simulink model "RefModel_compass_out2"  (R2019b)
settings: Solver=FixedStepDiscrete  StartTime=0.0  StopTime=35  FixedStep=0.1  RelTol=1e-3
values from neighbouring files (symbols this model uses):
  ax = double(typecast(uint8(temp),'single')')/1*1.0000000000    [V1000_decode_auto.m]
  ay = double(typecast(uint8(temp),'single')')/1*1.0000000000    [V1000_decode_auto.m]
  az = double(typecast(uint8(temp),'single')')/1*1.0000000000    [V1000_decode_auto.m]
  gx = double(typecast(uint8(temp),'single')')/1*1.0000000000    [V1000_decode_auto.m]
  gy = double(typecast(uint8(temp),'single')')/1*1.0000000000    [V1000_decode_auto.m]
  gz = double(typecast(uint8(temp),'single')')/1*1.0000000000    [V1000_decode_auto.m]
undefined symbols (not defined in the file or in its folder): ax_f, ay_f, az_f, gx_f, gy_f, gz_f, HD, mag2_xx, mag2_yx, mag2_zx, time_algo, time_imu, time_mag
libraries: simulink x1, aerolibgravity2 x1
settings Model: Creator=sl  LastModifiedBy=a4327
settings OptimizationCC: DefaultParameterBehavior=Inlined  UseDivisionForNetSlopeComputation=on  GainParamInheritBuiltInType=on  UseFloatMulNetSlope=on  InlineInvariantSignals=on  PassReuseOutputArgsAs=Individual arguments  ZeroExternalMemoryAtStartup=off  ZeroInternalMemoryAtStartup=off  NoFixptDivByZeroProtection=on  EfficientFloat2IntCast=on  LifeSpan=1  OptimizeBlockOrder=speed  DifferentSizesBufferReuse=on  EfficientTunableParamExpr=on
settings DebuggingCC: ParameterTunabilityLossMsg=error  ArithmeticOperatorsInVariantConditions=warning
settings HardwareCC: ProdBitPerPointer=32  ProdBitPerSizeT=32  ProdBitPerPtrDiffT=32  ProdLargestAtomicFloat=None  ProdWordSize=32  ProdLongLongMode=on  ProdHWDeviceType=Custom Processor->Custom Processor
settings SFSimCC: MATLABDynamicMemAlloc=off  CustomCodeUndefinedFunction=UseInterfaceOnly
settings RTWCC: SystemTargetFile=ert.tlc  TemplateMakefile=ert_default_tmf  GenerateReport=on  IncludeHyperlinkInReport=on  LaunchReport=on  GenerateTraceInfo=on  GenerateTraceReport=on  GenerateTraceReportSl=on  GenerateTraceReportSf=on  GenerateTraceReportEml=on  GenerateCodeMetricsReport=on
settings CodeAppCC: ForceParamTrailComments=on  IgnoreCustomStorageClasses=off  OperatorAnnotations=on  SimulinkDataObjDesc=on  SFDataObjDesc=on  CustomSymbolStrGlobalVar=rt$N$M  CustomSymbolStrType=$N$M  CustomSymbolStrFcn=$N$M$F  CustomSymbolStrMacro=$N$M  InsertBlockDesc=on
settings ERTTargetCC: TargetLangStandard=C99 (ISO)  GenerateSampleERTMain=on  IncludeMdlTerminateFcn=off  CombineSignalStateStructs=on  SupportAbsoluteTime=off  SupportComplex=off  SupportNonInlinedSFcns=on  InlinedParameterPlacement=NonHierarchical  ERTCustomFileTemplate=example_file_process.tlc  ERTFilePackagingFormat=CompactWithDataFile

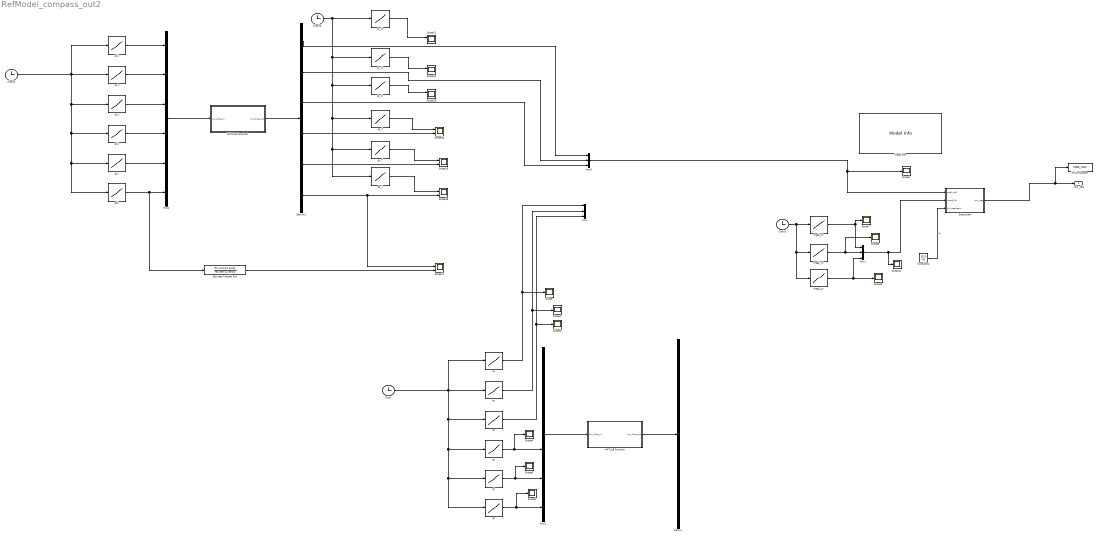
== system RefModel_compass_out2 ==
  Clock{,1..3} (4 alike) : Clock
  Constant2 : Constant  Value=[0 0 0]
  Demux : Demux  Outputs=6
  Demux1 : Demux  Outputs=6
  Discrete Transfer Fcn : DiscreteTransferFcn  Numerator=ftz.num{1:end}  Denominator=ftz.den{1:end}
  MATLAB Function : MATLAB Function  TreatAsAtomicUnit=on
  MATLAB Function1 : MATLAB Function  TreatAsAtomicUnit=on
  Model Info : simulink/Model-Wide Utilities/Model Info  Frame=on  DisplayStringWithTags=|  HorizontalTextAlignment=Left  LeftAlignmentValue=0.02
      | %<ModelVersion>
      | %<LastModificationDate>
      | 
      | Body Coordinate: forward - right - down
      | Navigation Coordinate: NED
      | 
      | input:
      | 	accB_ms2:  1x3  m/s^2
      | 	magB_Gs:   1x3  Gs
      | 	LLA_degdegm(lat,lon,height): 1x3 deg,deg,m  
      | output:
      | 	yaw_deg: 1x1 deg
  Mux : Mux  Inputs=3
  Mux1 : Mux  Inputs=3
  Mux2 : Mux  Inputs=6
  Mux3 : Mux  Inputs=3
  Mux4 : Mux  Inputs=6
  Scope{,1..10} (11 alike) : Scope
  Scope{11..17} (7 alike) : Scope  NumInputPorts=2
  Subsystem : Subsystem
  To Workspace : ToWorkspace  VariableName=MAG_YAW  SampleTime=-1
  ax : Lookup_n-D  NumberOfTableDimensions=1  BreakpointsForDimension1=time_imu  Table=ax  InternalRulePriority=Speed  RndMeth=Simplest  InputSameDT=on
  ax1 : Lookup_n-D  NumberOfTableDimensions=1  BreakpointsForDimension1=time_imu  Table=ax  InternalRulePriority=Speed  RndMeth=Simplest  InputSameDT=on
  ax_f1 : Lookup_n-D  NumberOfTableDimensions=1  BreakpointsForDimension1=time_algo  Table=ax_f  InternalRulePriority=Speed  RndMeth=Simplest  InputSameDT=on
  ay : Lookup_n-D  NumberOfTableDimensions=1  BreakpointsForDimension1=time_imu  Table=ay  InternalRulePriority=Speed  RndMeth=Simplest  InputSameDT=on
  ay1 : Lookup_n-D  NumberOfTableDimensions=1  BreakpointsForDimension1=time_imu  Table=ay  InternalRulePriority=Speed  RndMeth=Simplest  InputSameDT=on
  ay_f1 : Lookup_n-D  NumberOfTableDimensions=1  BreakpointsForDimension1=time_algo  Table=ay_f  InternalRulePriority=Speed  RndMeth=Simplest  InputSameDT=on
  az : Lookup_n-D  NumberOfTableDimensions=1  BreakpointsForDimension1=time_imu  Table=az  InternalRulePriority=Speed  RndMeth=Simplest  InputSameDT=on
  az1 : Lookup_n-D  NumberOfTableDimensions=1  BreakpointsForDimension1=time_imu  Table=az  InternalRulePriority=Speed  RndMeth=Simplest  InputSameDT=on
  az_f1 : Lookup_n-D  NumberOfTableDimensions=1  BreakpointsForDimension1=time_algo  Table=az_f  InternalRulePriority=Speed  RndMeth=Simplest  InputSameDT=on
  gx : Lookup_n-D  NumberOfTableDimensions=1  BreakpointsForDimension1=time_imu  Table=gx  InternalRulePriority=Speed  RndMeth=Simplest  InputSameDT=on
  gx1 : Lookup_n-D  NumberOfTableDimensions=1  BreakpointsForDimension1=time_imu  Table=gx  InternalRulePriority=Speed  RndMeth=Simplest  InputSameDT=on
  gx_f : Lookup_n-D  NumberOfTableDimensions=1  BreakpointsForDimension1=time_algo  Table=gx_f  InternalRulePriority=Speed  RndMeth=Simplest  InputSameDT=on
  gy : Lookup_n-D  NumberOfTableDimensions=1  BreakpointsForDimension1=time_imu  Table=gy  InternalRulePriority=Speed  RndMeth=Simplest  InputSameDT=on
  gy1 : Lookup_n-D  NumberOfTableDimensions=1  BreakpointsForDimension1=time_imu  Table=gy  InternalRulePriority=Speed  RndMeth=Simplest  InputSameDT=on
  gy_f : Lookup_n-D  NumberOfTableDimensions=1  BreakpointsForDimension1=time_algo  Table=gy_f  InternalRulePriority=Speed  RndMeth=Simplest  InputSameDT=on
  gz : Lookup_n-D  NumberOfTableDimensions=1  BreakpointsForDimension1=time_imu  Table=gz  InternalRulePriority=Speed  RndMeth=Simplest  InputSameDT=on
  gz1 : Lookup_n-D  NumberOfTableDimensions=1  BreakpointsForDimension1=time_imu  Table=gz  InternalRulePriority=Speed  RndMeth=Simplest  InputSameDT=on
  gz_f : Lookup_n-D  NumberOfTableDimensions=1  BreakpointsForDimension1=time_algo  Table=gz_f  InternalRulePriority=Speed  RndMeth=Simplest  InputSameDT=on
  mag2_xx : Lookup_n-D  NumberOfTableDimensions=1  BreakpointsForDimension1=time_mag  Table=mag2_xx  InternalRulePriority=Speed  RndMeth=Simplest  InputSameDT=on
  mag2_yx : Lookup_n-D  NumberOfTableDimensions=1  BreakpointsForDimension1=time_mag  Table=mag2_yx  InternalRulePriority=Speed  RndMeth=Simplest  InputSameDT=on
  mag2_zx : Lookup_n-D  NumberOfTableDimensions=1  BreakpointsForDimension1=time_mag  Table=mag2_zx  InternalRulePriority=Speed  RndMeth=Simplest  InputSameDT=on
  yaw_deg : Outport
  wires:
  Mux3/1 -> Scope1/1, Subsystem/1(accB_ms2)
  Constant2/1 -> Subsystem/3(LLA_degdegm)  "lla"
  Subsystem/1(yaw_deg) -> To Workspace/1, yaw_deg/1
  Clock1/1 -> mag2_zx/1, mag2_yx/1, mag2_xx/1
  gy/1 -> Scope5/1, Mux2/5
  gz/1 -> Scope6/1, Mux2/6
  Mux2/1 -> MATLAB Function/1(imu_filter_in)
  Clock/1 -> gz/1, gy/1, gx/1, az/1, ax/1, ay/1
  gx/1 -> Scope4/1, Mux2/4
  MATLAB Function/1(imu_filter_out) -> Demux/1
  mag2_yx/1 -> Scope8/1, Mux1/2
  mag2_xx/1 -> Scope7/1, Mux1/1
  mag2_zx/1 -> Scope9/1, Mux1/3
  Mux1/1 -> Scope10/1, Subsystem/2(magB_Gs)
  ax/1 -> Mux/1, Scope/1
  ay/1 -> Mux/2, Scope2/1
  az/1 -> Mux/3, Scope3/1
  gz_f/1 -> Scope16/1
  ay1/1 -> Mux4/2
  gx_f/1 -> Scope14/1
  ax1/1 -> Mux4/1
  Demux1/2 -> Mux3/2
  Clock3/1 -> gz_f/1, gy_f/1, gx_f/1, az_f1/1, ay_f1/1, ax_f1/1
  Demux1/6 -> Scope17/1, Scope16/2
  Demux1/5 -> Scope15/2
  Demux1/3 -> Mux3/3
  gy_f/1 -> Scope15/1
  Mux4/1 -> MATLAB Function1/1(imu_filter_in)
  ay_f1/1 -> Scope12/1
  gx1/1 -> Mux4/4
  Clock2/1 -> gz1/1, gy1/1, gx1/1, az1/1, ax1/1, ay1/1
  ax_f1/1 -> Scope11/1
  gz1/1 -> Discrete Transfer Fcn/1, Mux4/6
  Demux1/4 -> Scope14/2
  Demux1/1 -> Mux3/1
  az1/1 -> Mux4/3
  gy1/1 -> Mux4/5
  MATLAB Function1/1(imu_filter_out) -> Demux1/1
  az_f1/1 -> Scope13/1
  Discrete Transfer Fcn/1 -> Scope17/2

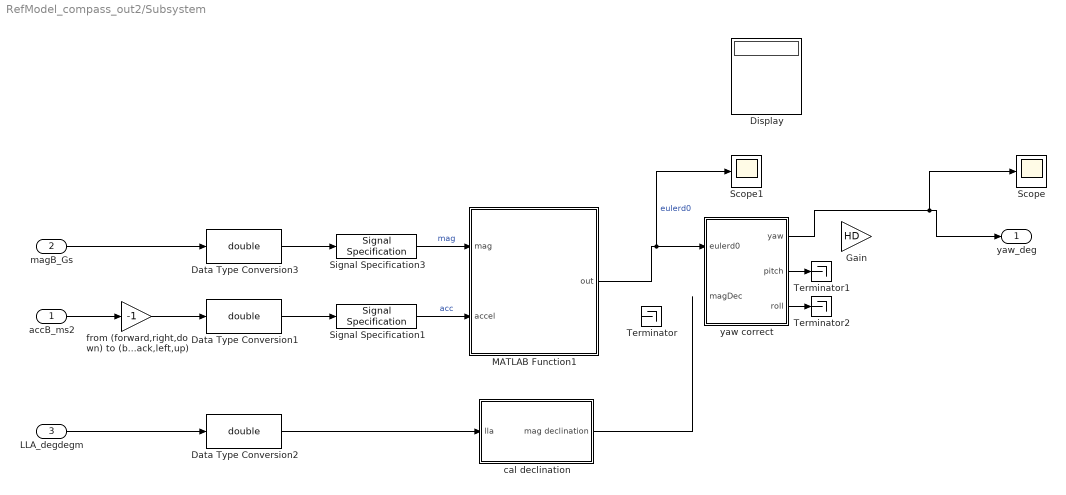
== system RefModel_compass_out2/Subsystem ==
  accB_ms2 : Inport  PortDimensions=[1,3]
  magB_Gs : Inport  Port=2  PortDimensions=[1,3]
  LLA_degdegm : Inport  Port=3  PortDimensions=[1,3]
  Data Type Conversion1 : DataTypeConversion  OutDataTypeStr=double
  Data Type Conversion2 : DataTypeConversion  OutDataTypeStr=double
  Data Type Conversion3 : DataTypeConversion  OutDataTypeStr=double
  Display : Display
  Gain : Gain  Gain=HD
  MATLAB Function1 : MATLAB Function  TreatAsAtomicUnit=on
  Scope : Scope
  Scope1 : Scope
  Signal Specification1 : SignalSpecification  Dimensions=[1,3]
  Signal Specification3 : SignalSpecification  Dimensions=[1,3]
  Terminator : Terminator
  Terminator1 : Terminator
  Terminator2 : Terminator
  cal declination : Subsystem
  from (forward,right,down) to (back,left,up) : Gain  Gain=-1
  yaw correct : Subsystem
  yaw_deg : Outport
  wires:
  from (forward,right,down) to (back,left,up)/1 -> Data Type Conversion1/1
  Signal Specification3/1 -> MATLAB Function1/1(mag)  "mag"
  yaw correct/2(pitch) -> Terminator1/1
  Data Type Conversion1/1 -> Signal Specification1/1
  Data Type Conversion3/1 -> Signal Specification3/1
  magB_Gs/1 -> Data Type Conversion3/1
  accB_ms2/1 -> from (forward,right,down) to (back,left,up)/1
  yaw correct/3(roll) -> Terminator2/1
  Signal Specification1/1 -> MATLAB Function1/2(accel)  "acc"
  cal declination/1(mag declination) -> ?
  Data Type Conversion2/1 -> cal declination/1(lla)
  LLA_degdegm/1 -> Data Type Conversion2/1
  MATLAB Function1/1(out) -> Scope1/1, yaw correct/1(eulerd0)  "eulerd0"
  yaw correct/1(yaw) -> Scope/1, yaw_deg/1

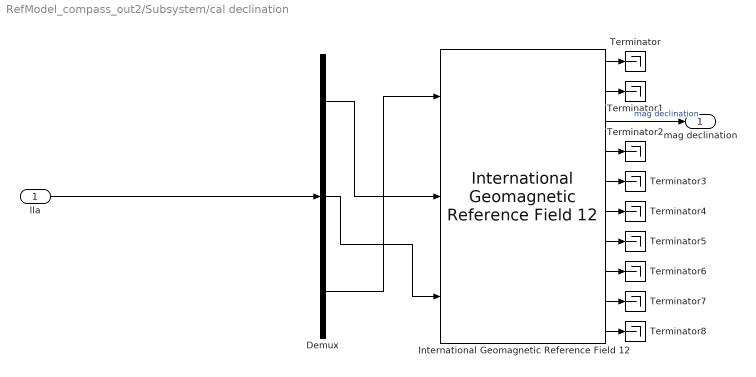
== system RefModel_compass_out2/Subsystem/cal declination ==
  lla : Inport
  Demux : Demux  Outputs=3
  International Geomagnetic Reference Field 12 : aerolibgravity2/International Geomagnetic Reference Field 12  units=Metric (MKS)  time_in=off  month=December  day=20  year=2019  action=None  sv_out=on
      settings: SourceProductName=Aerospace Blockset  SourceProductBaseCode=AE
  Terminator{,1..8} (9 alike) : Terminator
  mag declination : Outport
  wires:
  Demux/3 -> International Geomagnetic Reference Field 12/1
  Demux/1 -> International Geomagnetic Reference Field 12/2
  International Geomagnetic Reference Field 12/9 -> Terminator7/1
  International Geomagnetic Reference Field 12/10 -> Terminator8/1
  International Geomagnetic Reference Field 12/4 -> Terminator2/1
  International Geomagnetic Reference Field 12/1 -> Terminator/1
  Demux/2 -> International Geomagnetic Reference Field 12/3
  International Geomagnetic Reference Field 12/2 -> Terminator1/1
  International Geomagnetic Reference Field 12/3 -> mag declination/1  "mag declination"
  International Geomagnetic Reference Field 12/5 -> Terminator3/1
  International Geomagnetic Reference Field 12/6 -> Terminator4/1
  International Geomagnetic Reference Field 12/8 -> Terminator6/1
  International Geomagnetic Reference Field 12/7 -> Terminator5/1
  lla/1 -> Demux/1

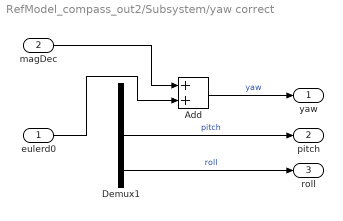
== system RefModel_compass_out2/Subsystem/yaw correct ==
  eulerd0 : Inport
  magDec : Inport  Port=2
  Add : Sum
  Demux1 : Demux  Outputs=3
  yaw : Outport
  pitch : Outport  Port=2
  roll : Outport  Port=3
  wires:
  magDec/1 -> Add/1
  Demux1/2 -> pitch/1  "pitch"
  Demux1/3 -> roll/1  "roll"
  eulerd0/1 -> Add/2
  Add/1 -> yaw/1  "yaw"

== matlab function RefModel_compass_out2/MATLAB Function1 ==
  data: imu_filter_in input; imu_filter_out output
function imu_filter_out = imu_filter(imu_filter_in)
% ftz.num{1:end}
% ftz.den{1:end}
% persistent
persistent imu_filter_in_buff
persistent imu_filter_out_buff
    if isempty(imu_filter_in_buff)
        imu_filter_in_buff = zeros(3,6);
    end
    if isempty(imu_filter_out_buff)
        imu_filter_out_buff = zeros(3,6);
    end 
    
    

imu_filter_in_buff(1,:)=imu_filter_in_buff(2,:);
imu_filter_in_buff(2,:)=imu_filter_in_buff(3,:);
imu_filter_in_buff(3,:)=imu_filter_in;
imu_filter_out_buff(1,:)=imu_filter_out_buff(2,:);
imu_filter_out_buff(2,:)=imu_filter_out_buff(3,:);
% imu_filter_out=imu_filter_in_buff(3,:)*0.1287+imu_filter_in_buff(2,:)*0.2574+imu_filter_in_buff(1,:)*0.1287-imu_filter_out_buff(2,:)*- 0.7613-imu_filter_out_buff(1,:)*0.276;
imu_filter_out=imu_filter_in_buff(3,:)*0.008771+imu_filter_in_buff(2,:)*0.01754+imu_filter_in_buff(1,:)*0.008771-imu_filter_out_buff(2,:)*- 1.718-imu_filter_out_buff(1,:)*0.7533;

imu_filter_out_buff(3,:)=imu_filter_out;

== matlab function RefModel_compass_out2/MATLAB Function ==
  data: imu_filter_in input; imu_filter_out output
function imu_filter_out = imu_filter(imu_filter_in)
% ftz.num{1:end}
% ftz.den{1:end}
% persistent
persistent imu_filter_in_buff
persistent imu_filter_out_buff
    if isempty(imu_filter_in_buff)
        imu_filter_in_buff = zeros(3,6);
    end
    if isempty(imu_filter_out_buff)
        imu_filter_out_buff = zeros(3,6);
    end 
    
    

imu_filter_in_buff(1,:)=imu_filter_in_buff(2,:);
imu_filter_in_buff(2,:)=imu_filter_in_buff(3,:);
imu_filter_in_buff(3,:)=imu_filter_in;
imu_filter_out_buff(1,:)=imu_filter_out_buff(2,:);
imu_filter_out_buff(2,:)=imu_filter_out_buff(3,:);
% imu_filter_out=imu_filter_in_buff(3,:)*0.1287+imu_filter_in_buff(2,:)*0.2574+imu_filter_in_buff(1,:)*0.1287-imu_filter_out_buff(2,:)*- 0.7613-imu_filter_out_buff(1,:)*0.276;
imu_filter_out=imu_filter_in_buff(3,:)*0.008771+imu_filter_in_buff(2,:)*0.01754+imu_filter_in_buff(1,:)*0.008771-imu_filter_out_buff(2,:)*- 1.718-imu_filter_out_buff(1,:)*0.7533;

imu_filter_out_buff(3,:)=imu_filter_out;

== matlab function RefModel_compass_out2/Subsystem/MATLAB Function1 ==
  data: mag input; accel input; out output
function out  = compass(mag,accel)
    quat0 = zeros(1,4);
    eulerd0 = zeros(1,3);
    temp=ecompass(accel,mag);
    quat0 = compact(temp);
     eulerd0 = eulerd(quat0);
%     eulerd0 = to_euler(quat0);
    out=eulerd0(1);
    
    
%     out=atan2(mag(2),mag(1));
    if out<0
    out=out+2*pi;
    end
    out=out*180/pi;
end


function eout = eulerd(quat)
% rotate 'ZYX'
qa = quat(1);
qb = quat(2);
qc = quat(3);
qd = quat(4);
the1 = 1;
the2 = 2;

tmp = qb.*qd.*the2 - qa.*qc.*the2;
if tmp > the1
    tmp = the1;
elseif tmp < -the1
    tmp = -the1;
end
% tmp(tmp > the1) = the1;
% tmp(tmp < -the1) = -the1;
b = -asin(tmp);
a = atan2((qa.*qd.*the2 + qb.*qc.*the2),(qa.^2.*the2 - the1 + qb.^2.*the2));
c = atan2((qa.*qb.*the2 + qc.*qd.*the2),(qa.^2.*the2 - the1 + qd.^2.*the2));
eout = [a b c];
end
% 
% function [eulerd0,quat0] = compass(i,accel,mag,imuUpdateFs,magUpdateFs)
%     fs = imuUpdateFs;
%     quat0 = zeros(1,4);
%     eulerd0 = zeros(1,3);
%     if rem(i,fs/magUpdateFs) == 0 && i ~= 1
%         quat0 = compact(ecompass(accel,mag));
%         eulerd0 = eulerd(quat0);
%     end
% end
